simulink model "motor_cc_velocidade_cont_PID"  (R2019b)
settings: Solver=VariableStepAuto  StartTime=0.0  StopTime=5  RelTol=1e-3
values from neighbouring files (symbols this model uses):
  b = 0.1    [motor.m]
  J = 0.01    [motor.m]
  Ke = 0.01    [motor.m]
  Kt = 0.01    [motor.m]
  L = 0.5    [motor.m]
  R = 1    [motor.m]
settings Model: Creator=fernandopassold  LastModifiedBy=fernandopassold
settings DataIOCC: ReturnWorkspaceOutputs=off
settings DebuggingCC: ArithmeticOperatorsInVariantConditions=warning
settings SFSimCC: SimUseLocalCustomCode=off  CustomCodeUndefinedFunction=UseInterfaceOnly
settings RTWCC: RTWUseLocalCustomCode=off

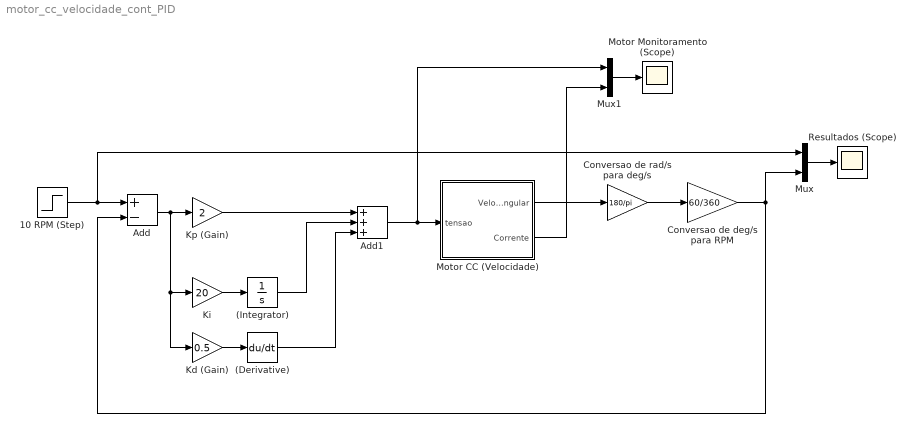
== system motor_cc_velocidade_cont_PID ==
  (Derivative) : Derivative
  (Integrator) : Integrator
  10 RPM (Step) : Step  After=10  SampleTime=0
  Add : Sum  Inputs=+-
  Add1 : Sum  Inputs=+++
  Conversao de deg/s para RPM : Gain  Gain=60/360
  Conversao de rad/s para deg/s : Gain  Gain=180/pi
  Kd (Gain) : Gain  Gain=0.5
  Ki : Gain  Gain=20
  Kp (Gain) : Gain  Gain=2
  Motor Monitoramento (Scope) : Scope
  Motor CC (Velocidade) : Subsystem
  Mux : Mux  Inputs=2
  Mux1 : Mux  Inputs=2
  Resultados (Scope) : Scope
  wires:
  Motor CC (Velocidade)/1(Velocidade Angular) -> Conversao de rad/s para deg/s/1
  Conversao de rad/s para deg/s/1 -> Conversao de deg/s para RPM/1
  Add/1 -> Ki/1, Kd (Gain)/1, Kp (Gain)/1
  10 RPM (Step)/1 -> Mux/1, Add/1
  Conversao de deg/s para RPM/1 -> Mux/2, Add/2
  Mux/1 -> Resultados (Scope)/1
  Motor CC (Velocidade)/2(Corrente) -> Mux1/2
  Mux1/1 -> Motor Monitoramento (Scope)/1
  Kd (Gain)/1 -> (Derivative)/1
  Add1/1 -> Mux1/1, Motor CC (Velocidade)/1(tensao)
  Kp (Gain)/1 -> Add1/1
  (Derivative)/1 -> Add1/3
  Ki/1 -> (Integrator)/1
  (Integrator)/1 -> Add1/2

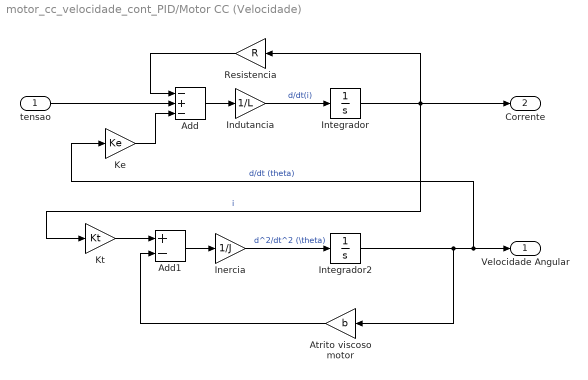
== system motor_cc_velocidade_cont_PID/Motor CC (Velocidade) ==
  tensao : Inport
  Add : Sum  Inputs=-+-
  Add1 : Sum  Inputs=+-
  Atrito viscoso motor : Gain  Gain=b
  Indutancia : Gain  Gain=1/L
  Inercia : Gain  Gain=1/J
  Integrador : Integrator
  Integrador2 : Integrator
  Ke : Gain  Gain=Ke
  Kt : Gain  Gain=Kt
  Resistencia : Gain  Gain=R
  Velocidade Angular : Outport  VectorParamsAs1DForOutWhenUnconnected=off
  Corrente : Outport  Port=2  VectorParamsAs1DForOutWhenUnconnected=off
  wires:
  Ke/1 -> Add/3
  Add1/1 -> Inercia/1
  Inercia/1 -> Integrador2/1  "d^2/dt^2 (\\theta)"
  Add/1 -> Indutancia/1
  tensao/1 -> Add/2
  Indutancia/1 -> Integrador/1  "d/dt(i)"
  Integrador2/1 -> Velocidade Angular/1, Ke/1, Atrito viscoso motor/1  "d/dt (theta)"
  Atrito viscoso motor/1 -> Add1/2
  Kt/1 -> Add1/1
  Integrador/1 -> Corrente/1, Kt/1, Resistencia/1  "i"
  Resistencia/1 -> Add/1
